simulink model "conver_meter_to_feet"  (R2021a)
settings: Solver=VariableStepAuto  StartTime=0.0  StopTime=10.0  RelTol=1e-3
settings Model: Creator=HP  LastModifiedBy=HP

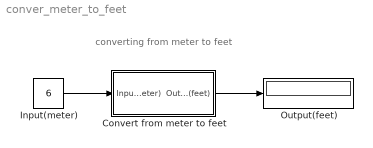
== system conver_meter_to_feet ==
  note: converting from meter to feet
  " Input(meter)" : Constant  Value=6
  Convert from meter to feet : Subsystem
  Output(feet) : Display
  wires:
  " Input(meter)"/1 -> Convert from meter to feet/1(Input(meter))
  Convert from meter to feet/1(Output(feet)) -> Output(feet)/1

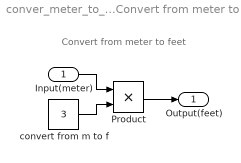
== system conver_meter_to_feet/Convert from meter to feet ==
  note: Convert from meter to feet
  Input(meter) : Inport
  Product : Product
  convert from m to f : Constant  Value=3
  Output(feet) : Outport
  wires:
  Product/1 -> Output(feet)/1
  convert from m to f/1 -> Product/2
  Input(meter)/1 -> Product/1
